simulink model "PID_test"  (R2021a)
settings: Solver=FixedStepAuto  StartTime=0.0  StopTime=inf  RelTol=1e-3
undefined symbols (not defined in the file or in its folder): AccelerationOrForce, TypeMask, Yaw
libraries: robotlib x2
settings Model: Creator=esl  LastModifiedBy=esl
settings OptimizationCC: UseDivisionForNetSlopeComputation=on  GainParamInheritBuiltInType=on  UseFloatMulNetSlope=on  EnhancedBackFolding=on  PassReuseOutputArgsAs=Individual arguments  ZeroExternalMemoryAtStartup=off  ZeroInternalMemoryAtStartup=off  EfficientFloat2IntCast=on  MaxStackSize=64  OptimizeBlockOrder=speed  DifferentSizesBufferReuse=on  OptimizationCustomize=off  EfficientTunableParamExpr=on
settings DebuggingCC: ParameterTunabilityLossMsg=error
settings HardwareCC: ProdBitPerLong=64  ProdHWDeviceType=Intel->x86-64 (Linux 64)  UseEmbeddedCoderFeatures=off
settings SFSimCC: MATLABDynamicMemAlloc=off
settings RTWCC: SystemTargetFile=ert.tlc  HardwareBoard=Robot Operating System (ROS)  TLCOptions="-aInlineSetEventsForThisBaseRateFcn=TLC_FALSE -aSuppressMultiTaskScheduler=TLC_FALSE  -aRateBasedStepFcn=0"  TemplateMakefile=ert_default_tmf  GenerateReport=on  Toolchain=Catkin  LaunchReport=on  TargetLang=C++
settings CodeAppCC: ForceParamTrailComments=on  IgnoreCustomStorageClasses=off  OperatorAnnotations=on  SimulinkDataObjDesc=on  SFDataObjDesc=on  InsertBlockDesc=on
settings ERTTargetCC: CodeInterfacePackaging=C++ class  SupportNonInlinedSFcns=on  RootIOFormat=Structure reference

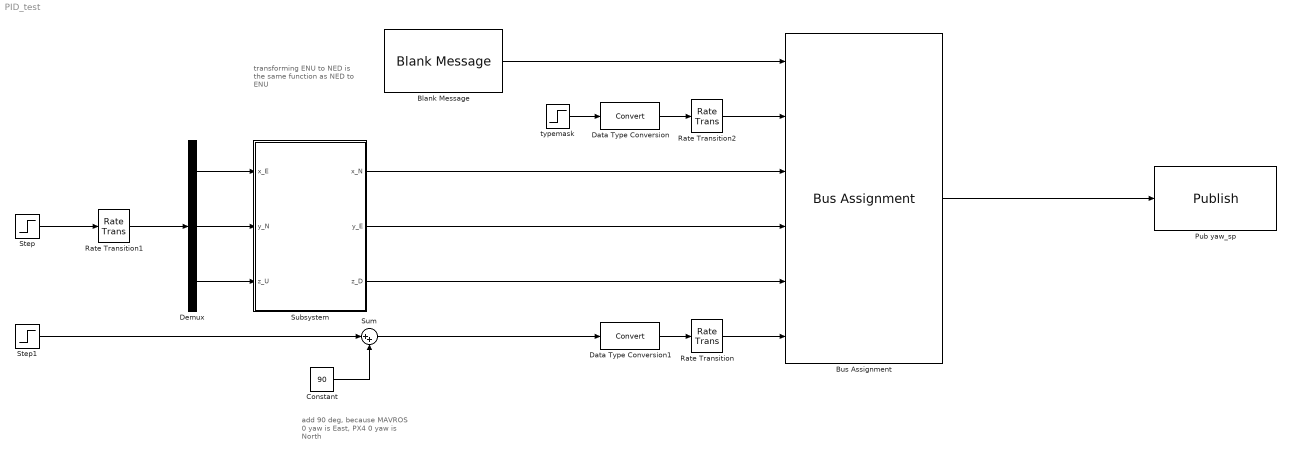
== system PID_test ==
  note: transforming
      | ENU to NED
      | is the same function as
      | NED to ENU
  note: add 90 deg, because
      | MAVROS 0 yaw is East,
      | PX4 0 yaw is North
  Blank Message : robotlib/Blank Message  messageClass=Message  entityType=mavros_msgs/PositionTarget  messageType=mavros_msgs/PositionTarget  SampleTime=inf  legacyBusStruct=off
  Bus Assignment : BusAssignment  AssignedSignals=TypeMask,AccelerationOrForce.X,AccelerationOrForce.Y,AccelerationOrForce.Z,Yaw
  Constant : Constant  Value=90
  Data Type Conversion : DataTypeConversion
  Data Type Conversion1 : DataTypeConversion
  Demux : Demux  Outputs=3
  Pub yaw_sp : robotlib/Publish  topicSource=Select from ROS network  topic=/mavros/setpoint_raw/local  messageType=mavros_msgs/PositionTarget  legacyBusStruct=off  messageQueueLength=1
  Rate Transition : RateTransition  OutPortSampleTime=0.03
  Rate Transition1 : RateTransition  OutPortSampleTime=0.03
  Rate Transition2 : RateTransition  OutPortSampleTime=0.03
  Step : Step  After=[0 0 0]  SampleTime=0
  Step1 : Step  After=0  SampleTime=0
  Subsystem : Subsystem
  Sum : Sum  Inputs=|++
  typemask : Step  Time=0  After=2111  OutDataTypeStr=single  SampleTime=0
  wires:
  Sum/1 -> Data Type Conversion1/1
  Rate Transition/1 -> Bus Assignment/6
  Data Type Conversion/1 -> Rate Transition2/1
  Data Type Conversion1/1 -> Rate Transition/1
  Rate Transition2/1 -> Bus Assignment/2
  typemask/1 -> Data Type Conversion/1
  Step/1 -> Rate Transition1/1
  Step1/1 -> Sum/1
  Bus Assignment/1 -> Pub yaw_sp/1
  Blank Message/1 -> Bus Assignment/1
  Rate Transition1/1 -> Demux/1
  Constant/1 -> Sum/2
  Demux/1 -> Subsystem/1(x_E)
  Demux/2 -> Subsystem/2(y_N)
  Demux/3 -> Subsystem/3(z_U)
  Subsystem/1(x_N) -> Bus Assignment/3
  Subsystem/2(y_E) -> Bus Assignment/4
  Subsystem/3(z_D) -> Bus Assignment/5

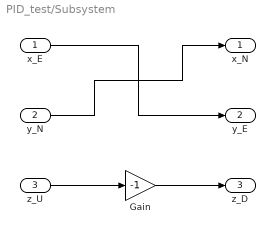
== system PID_test/Subsystem ==
  x_E : Inport
  y_N : Inport  Port=2
  z_U : Inport  Port=3
  Gain : Gain  Gain=-1
  x_N : Outport
  y_E : Outport  Port=2
  z_D : Outport  Port=3
  wires:
  y_N/1 -> x_N/1
  x_E/1 -> y_E/1
  Gain/1 -> z_D/1
  z_U/1 -> Gain/1
